simulink model "YawModel"  (R2013a)
settings: Solver=ode45  StartTime=0.0  StopTime=30  RelTol=1e-3
values from neighbouring files (symbols this model uses):
  omega_0 = 1.7    [Height_Controller_PID.m]    (also in Yaw_PD.m = 520)
undefined symbols (not defined in the file or in its folder): D, I_Psi, J, Kw, Motor_TimeConstant, Speed_yIntercept
libraries: simulink x3
settings Model: Creator=Ross  LastModifiedBy=Ross

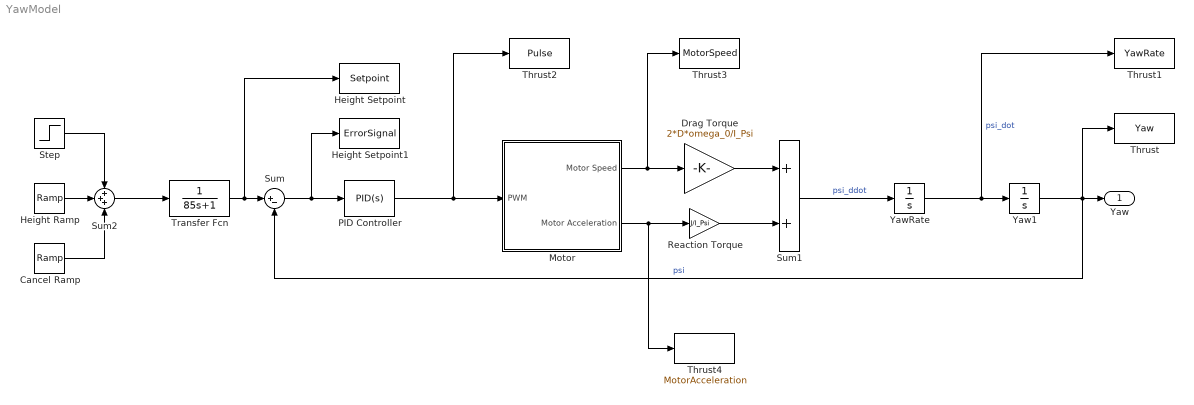
== system YawModel ==
  Cancel Ramp : simulink/Sources/Ramp  slope=-1  start=5  X0=0
  Drag Torque : Gain  Gain=2*D*omega_0/I_Psi
  Height Ramp : simulink/Sources/Ramp  slope=1  start=1  X0=0
  Height Setpoint : ToWorkspace  VariableName=Setpoint  SampleTime=-1  SaveFormat=Timeseries
  Height Setpoint1 : ToWorkspace  VariableName=ErrorSignal  SampleTime=-1  SaveFormat=Timeseries
  Motor : Subsystem
  PID Controller : simulink/Continuous/PID Controller  Controller=PID  TimeDomain=Continuous-time  SampleTime=1  IntegratorMethod=Forward Euler  FilterMethod=Forward Euler  Form=Parallel  P=3310  I=2613  D=1047  N=100  InitialConditionSource=internal  InitialConditionForIntegrator=0  InitialConditionForFilter=0  ExternalReset=none  LimitOutput=off  UpperSaturationLimit=2  LowerSaturationLimit=0  LinearizeAsGain=on  AntiWindupMode=clamping  Kb=1  TrackingMode=off  Kt=1  PParamMin=[]  PParamMax=[]  IParamMin=[]  IParamMax=[]  DParamMin=[]  DParamMax=[]  NParamMin=[]  NParamMax=[]  KbParamMin=[]  KbParamMax=[]  KtParamMin=[]  KtParamMax=[]  POutMin=[]  POutMax=[]  IOutMin=[]  IOutMax=[]  DOutMin=[]  DOutMax=[]  NOutMin=[]  NOutMax=[]  KbOutMin=[]  KbOutMax=[]  KtOutMin=[]  KtOutMax=[]  IntegratorOutMin=[]  IntegratorOutMax=[]  FilterOutMin=[]  FilterOutMax=[]  SumOutMin=[]  SumOutMax=[]  SumI1OutMin=[]  SumI1OutMax=[]  SumI2OutMin=[]  SumI2OutMax=[]  SumI3OutMin=[]  SumI3OutMax=[]  SumDOutMin=[]  SumDOutMax=[]  SaturationOutMin=[]  SaturationOutMax=[]  IntegratorContinuousStateAttributes=''  IntegratorStateMustResolveToSignalObject=off  IntegratorRTWStateStorageClass=Auto  FilterContinuousStateAttributes=''  FilterStateMustResolveToSignalObject=off  FilterRTWStateStorageClass=Auto
  Reaction Torque : Gain  Gain=J/I_Psi
  Step : Step  Time=10  SampleTime=0
  Sum : Sum  Inputs=|+-
  Sum1 : Sum
  Sum2 : Sum  Inputs=+++
  Thrust : ToWorkspace  VariableName=Yaw  SampleTime=-1  SaveFormat=Timeseries
  Thrust1 : ToWorkspace  VariableName=YawRate  SampleTime=-1  SaveFormat=Timeseries
  Thrust2 : ToWorkspace  VariableName=Pulse  SampleTime=-1  SaveFormat=Timeseries
  Thrust3 : ToWorkspace  VariableName=MotorSpeed  SampleTime=-1  SaveFormat=Timeseries
  Thrust4 : ToWorkspace  VariableName=MotorAcceleration  SampleTime=-1  SaveFormat=Timeseries
  Transfer Fcn : TransferFcn  Denominator=[85 1]
  Yaw1 : Integrator  LowerSaturationLimit=0
  YawRate : Integrator
  Yaw : Outport
  wires:
  Yaw1/1 -> Sum/2, Thrust/1, Yaw/1  "psi"
  YawRate/1 -> Thrust1/1, Yaw1/1  "psi_dot"
  Sum1/1 -> YawRate/1  "psi_ddot"
  Motor/2(Motor Acceleration) -> Thrust4/1, Reaction Torque/1
  Drag Torque/1 -> Sum1/1
  Reaction Torque/1 -> Sum1/2
  Step/1 -> Sum2/1
  Height Ramp/1 -> Sum2/2
  Cancel Ramp/1 -> Sum2/3
  Sum2/1 -> Transfer Fcn/1
  Sum/1 -> Height Setpoint1/1, PID Controller/1
  Motor/1(Motor Speed) -> Drag Torque/1, Thrust3/1
  PID Controller/1 -> Motor/1(PWM), Thrust2/1
  Transfer Fcn/1 -> Height Setpoint/1, Sum/1

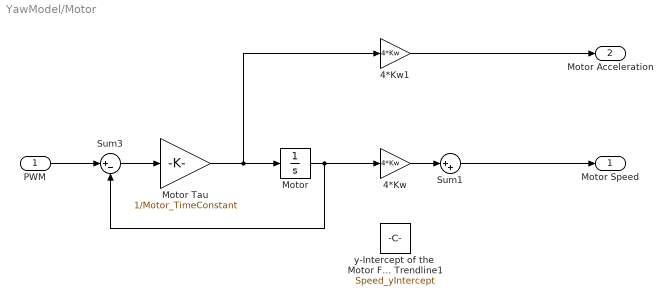
== system YawModel/Motor ==
  PWM : Inport
  4*Kw : Gain  Gain=4*Kw
  4*Kw1 : Gain  Gain=4*Kw
  Motor : Integrator
  Motor Tau : Gain  Gain=1/Motor_TimeConstant
  Sum1 : Sum  Inputs=|++
  Sum3 : Sum  Inputs=|+-
  y-Intercept of the  Motor Forc Trendline1 : Constant  Value=Speed_yIntercept
  Motor Speed : Outport
  Motor Acceleration : Outport  Port=2
  wires:
  Motor Tau/1 -> 4*Kw1/1, Motor/1
  Motor/1 -> 4*Kw/1, Sum3/2
  PWM/1 -> Sum3/1
  Sum3/1 -> Motor Tau/1
  4*Kw/1 -> Sum1/1
  Sum1/1 -> Motor Speed/1
  4*Kw1/1 -> Motor Acceleration/1
